simulink model "Model_silnika_mdl2"  (Simulink 9.1)
settings: Solver=ode45  StartTime=0.0  StopTime=100  FixedStep=1  RelTol=1e-8  EnableMultiTasking=on
values from neighbouring files (symbols this model uses):
  G = 4.2    [net_opuznienie_30.mat]    (also in parametrySilnika.m)
  G1 = 4.2    [net_opuznienie_30.mat]    (also in parametrySilnika.m)
  J = 1    [net_opuznienie_30.mat]    (also in parametrySilnika.m)
  J1 = 1.3    [net_opuznienie_30.mat]    (also in parametrySilnika.m = 1)
  Lt = 46    [net_opuznienie_30.mat]    (also in parametrySilnika.m)
  Lt1 = 59.8    [net_opuznienie_30.mat]    (also in parametrySilnika.m = 69)
  Lw = 125    [net_opuznienie_30.mat]    (also in parametrySilnika.m)
  Lw1 = 162.5    [net_opuznienie_30.mat]    (also in parametrySilnika.m = 125)
  Rt = 5    [net_opuznienie_30.mat]    (also in parametrySilnika.m)
  Rt1 = 5    [net_opuznienie_30.mat]    (also in parametrySilnika.m)
undefined symbols (not defined in the file or in its folder): sigbuilder_block
libraries: simulink x2
settings Model: Creator=zen  LastModifiedBy=Szwank
settings DataIOCC: LimitDataPoints=on  SignalLoggingSaveFormat=ModelDataLogs
settings OptimizationCC: ExpressionDepthLimit=2147483647  InitFltsAndDblsToZero=on
settings DebuggingCC: SaveWithParameterizedLinksMsg=none  SignalResolutionControl=TryResolveAllWithWarning  SolverPrmCheckMsg=warning  MultiTaskDSMMsg=warning  MultiTaskCondExecSysMsg=none  FcnCallInpInsideContextMsg=warning  StateNameClashWarn=warning
settings GRTTargetCC: TargetFcnLib=ansi_tfl_tmw.mat  GeneratePreprocessorConditionals=Disable all

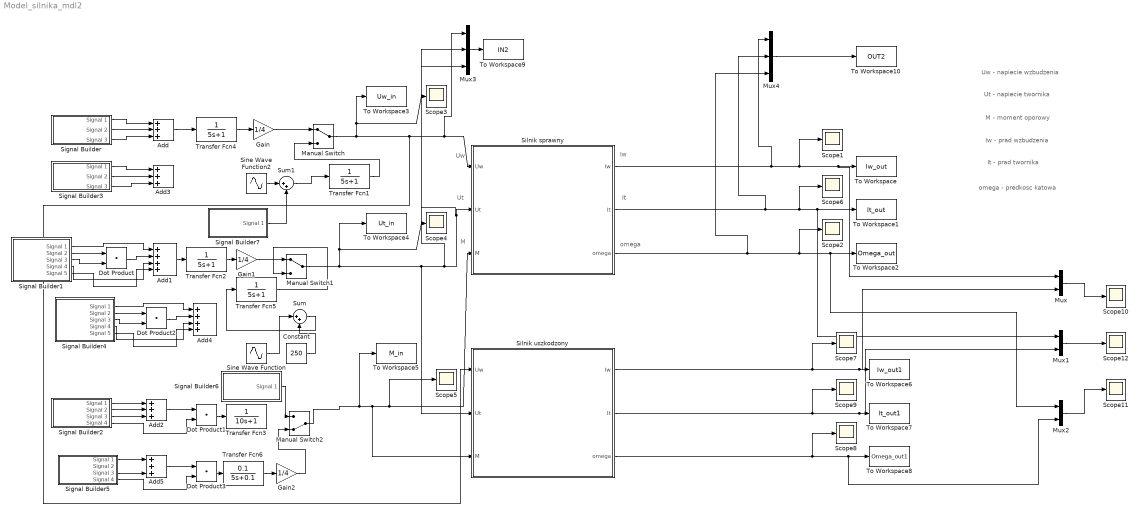
== system Model_silnika_mdl2 ==
  note: Uw
  note: Ut
  note: M
  note: Iw
  note: It
  note: omega
  note: Uw - napiecie wzbudzenia
  note: Ut - napiecie twornika
  note: M - moment oporowy
  note: Iw - prad wzbudzenia
  note: It - prad twornika
  note: omega - predkosc katowa
  Add{,2..3,5} (4 alike) : Sum  Inputs=+++
  Add1 : Sum  Inputs=++++
  Add4 : Sum  Inputs=++++
  Constant : Constant  Value=250
  Dot Product{,1..3} (4 alike) : DotProduct  InputSameDT=on  OutDataTypeStr=Inherit: Inherit via internal rule
  Gain : Gain  Gain=1/4
  Gain1 : Gain  Gain=1/4
  Gain2 : Gain  Gain=1/4
  Manual Switch : ManualSwitch
  Manual Switch1 : ManualSwitch
  Manual Switch2 : ManualSwitch  CurrentSetting=0
  Mux : Mux  Inputs=2
  Mux1 : Mux  Inputs=2
  Mux2 : Mux  Inputs=2
  Mux3 : Mux  Inputs=3
  Mux4 : Mux  Inputs=3
  Scope{1..12} (12 alike) : Scope
  Signal Builder : Subsystem  Tag=STV Subsys  LoadFcn=sigbuilder_block('load');  StartFcn=sigbuilder_block('start');  StopFcn=sigbuilder_block('stop');  ClipboardFcn=sigbuilder_block('clipboard');  mask(Sigbuilder block){tuvar=[0:10]}
      mask help: Create and generate interchangeable groups of signals whose waveforms are piecewise linear.
      mask init:
      | if ~strcmp(get_param(bdroot(gcbh),'SimulationStatus'),'stopped') tuvar = sigbuilder_block('maskInit'); end
      settings: CopyFcn=sigbuilder_block('copy');  DeleteFcn=sigbuilder_block('delete');  ModelCloseFcn=sigbuilder_block('modelClose');  PreSaveFcn=sigbuilder_block('preSave');  PauseFcn=sigbuilder_block('pause')  ContinueFcn=sigbuilder_block('continue')  NameChangeFcn=sigbuilder_block('namechange');  OpenFcn=sigbuilder_block('open',[159 116.25 948 506.25 ]);  CloseFcn=sigbuilder_block('close');
      mask Display: plot(0, 0, 100, 100,[2, 2, 32, 32, 2], [68, 8, 8, 68, 68],[32, 2], [38, 38], [32, 19, 2],[53, 60, 44], [32, 17, 17, 2],[16, 16, 31, 31]);txt = getActiveGroup(gcbh);text(2, 100, txt,'verticalAlignment', 'top');
  Signal Builder1 : Subsystem  Tag=STV Subsys  LoadFcn=sigbuilder_block('load');  StartFcn=sigbuilder_block('start');  StopFcn=sigbuilder_block('stop');  ClipboardFcn=sigbuilder_block('clipboard');  mask(Sigbuilder block){tuvar=[0:10]}
      mask help: Create and generate interchangeable groups of signals whose waveforms are piecewise linear.
      mask init:
      | if ~strcmp(get_param(bdroot(gcbh),'SimulationStatus'),'stopped') tuvar = sigbuilder_block('maskInit'); end
      settings: CopyFcn=sigbuilder_block('copy');  DeleteFcn=sigbuilder_block('delete');  ModelCloseFcn=sigbuilder_block('modelClose');  PreSaveFcn=sigbuilder_block('preSave');  PauseFcn=sigbuilder_block('pause')  ContinueFcn=sigbuilder_block('continue')  NameChangeFcn=sigbuilder_block('namechange');  OpenFcn=sigbuilder_block('open',[49.5 13.5 1254 711.75 ]);  CloseFcn=sigbuilder_block('close');
      mask Display: plot(0, 0, 100, 100,[2, 2, 32, 32, 2], [68, 8, 8, 68, 68],[32, 2], [38, 38], [32, 19, 2],[53, 60, 44], [32, 17, 17, 2],[16, 16, 31, 31]);txt = getActiveGroup(gcbh);text(2, 100, txt,'verticalAlignment', 'top');
  Signal Builder2 : Subsystem  Tag=STV Subsys  LoadFcn=sigbuilder_block('load');  StartFcn=sigbuilder_block('start');  StopFcn=sigbuilder_block('stop');  ClipboardFcn=sigbuilder_block('clipboard');  mask(Sigbuilder block){tuvar=[0:10]}
      mask help: Create and generate interchangeable groups of signals whose waveforms are piecewise linear.
      mask init:
      | if ~strcmp(get_param(bdroot(gcbh),'SimulationStatus'),'stopped') tuvar = sigbuilder_block('maskInit'); end
      settings: CopyFcn=sigbuilder_block('copy');  DeleteFcn=sigbuilder_block('delete');  ModelCloseFcn=sigbuilder_block('modelClose');  PreSaveFcn=sigbuilder_block('preSave');  PauseFcn=sigbuilder_block('pause')  ContinueFcn=sigbuilder_block('continue')  NameChangeFcn=sigbuilder_block('namechange');  OpenFcn=sigbuilder_block('open',[6 6 948 531 ]);  CloseFcn=sigbuilder_block('close');
      mask Display: plot(0, 0, 100, 100,[2, 2, 32, 32, 2], [68, 8, 8, 68, 68],[32, 2], [38, 38], [32, 19, 2],[53, 60, 44], [32, 17, 17, 2],[16, 16, 31, 31]);txt = getActiveGroup(gcbh);text(2, 100, txt,'verticalAlignment', 'top');
  Signal Builder3 : Subsystem  Tag=STV Subsys  LoadFcn=sigbuilder_block('load');  StartFcn=sigbuilder_block('start');  StopFcn=sigbuilder_block('stop');  ClipboardFcn=sigbuilder_block('clipboard');  mask(Sigbuilder block){tuvar=[0:10]}
      mask help: Create and generate interchangeable groups of signals whose waveforms are piecewise linear.
      mask init:
      | if ~strcmp(get_param(bdroot(gcbh),'SimulationStatus'),'stopped') tuvar = sigbuilder_block('maskInit'); end
      settings: CopyFcn=sigbuilder_block('copy');  DeleteFcn=sigbuilder_block('delete');  ModelCloseFcn=sigbuilder_block('modelClose');  PreSaveFcn=sigbuilder_block('preSave');  PauseFcn=sigbuilder_block('pause')  ContinueFcn=sigbuilder_block('continue')  NameChangeFcn=sigbuilder_block('namechange');  OpenFcn=sigbuilder_block('open',[6 30.75 948 506.25 ]);  CloseFcn=sigbuilder_block('close');
      mask Display: plot(0, 0, 100, 100,[2, 2, 32, 32, 2], [68, 8, 8, 68, 68],[32, 2], [38, 38], [32, 19, 2],[53, 60, 44], [32, 17, 17, 2],[16, 16, 31, 31]);txt = getActiveGroup(gcbh);text(2, 100, txt,'verticalAlignment', 'top');
  Signal Builder4 : Subsystem  Tag=STV Subsys  LoadFcn=sigbuilder_block('load');  StartFcn=sigbuilder_block('start');  StopFcn=sigbuilder_block('stop');  ClipboardFcn=sigbuilder_block('clipboard');  mask(Sigbuilder block){tuvar=[0:10]}
      mask help: Create and generate interchangeable groups of signals whose waveforms are piecewise linear.
      mask init:
      | if ~strcmp(get_param(bdroot(gcbh),'SimulationStatus'),'stopped') tuvar = sigbuilder_block('maskInit'); end
      settings: CopyFcn=sigbuilder_block('copy');  DeleteFcn=sigbuilder_block('delete');  ModelCloseFcn=sigbuilder_block('modelClose');  PreSaveFcn=sigbuilder_block('preSave');  PauseFcn=sigbuilder_block('pause')  ContinueFcn=sigbuilder_block('continue')  NameChangeFcn=sigbuilder_block('namechange');  OpenFcn=sigbuilder_block('open',[196.5 116.25 948 526.5 ]);  CloseFcn=sigbuilder_block('close');
      mask Display: plot(0, 0, 100, 100,[2, 2, 32, 32, 2], [68, 8, 8, 68, 68],[32, 2], [38, 38], [32, 19, 2],[53, 60, 44], [32, 17, 17, 2],[16, 16, 31, 31]);txt = getActiveGroup(gcbh);text(2, 100, txt,'verticalAlignment', 'top');
  Signal Builder5 : Subsystem  Tag=STV Subsys  LoadFcn=sigbuilder_block('load');  StartFcn=sigbuilder_block('start');  StopFcn=sigbuilder_block('stop');  ClipboardFcn=sigbuilder_block('clipboard');  mask(Sigbuilder block){tuvar=[0:10]}
      mask help: Create and generate interchangeable groups of signals whose waveforms are piecewise linear.
      mask init:
      | if ~strcmp(get_param(bdroot(gcbh),'SimulationStatus'),'stopped') tuvar = sigbuilder_block('maskInit'); end
      settings: CopyFcn=sigbuilder_block('copy');  DeleteFcn=sigbuilder_block('delete');  ModelCloseFcn=sigbuilder_block('modelClose');  PreSaveFcn=sigbuilder_block('preSave');  PauseFcn=sigbuilder_block('pause')  ContinueFcn=sigbuilder_block('continue')  NameChangeFcn=sigbuilder_block('namechange');  OpenFcn=sigbuilder_block('open',[57 31.5 948 531 ]);  CloseFcn=sigbuilder_block('close');
      mask Display: plot(0, 0, 100, 100,[2, 2, 32, 32, 2], [68, 8, 8, 68, 68],[32, 2], [38, 38], [32, 19, 2],[53, 60, 44], [32, 17, 17, 2],[16, 16, 31, 31]);txt = getActiveGroup(gcbh);text(2, 100, txt,'verticalAlignment', 'top');
  Signal Builder6 : Subsystem  Tag=STV Subsys  LoadFcn=sigbuilder_block('load');  StartFcn=sigbuilder_block('start');  StopFcn=sigbuilder_block('stop');  ClipboardFcn=sigbuilder_block('clipboard');  mask(Sigbuilder block){tuvar=[0:10]}
      mask help: Simulink:masks:SigbuilderBlock_MD
      mask init:
      | if ~strcmp(get_param(bdroot(gcbh),'SimulationStatus'),'stopped') tuvar = sigbuilder_block('maskInit'); end
      settings: CopyFcn=sigbuilder_block('copy');  DeleteFcn=sigbuilder_block('delete');  ModelCloseFcn=sigbuilder_block('modelClose');  PreSaveFcn=sigbuilder_block('preSave');  PauseFcn=sigbuilder_block('pause');  ContinueFcn=sigbuilder_block('continue');  NameChangeFcn=sigbuilder_block('namechange');  OpenFcn=sigbuilder_block('open',[437.6 199.2 550.4 400 ]);  CloseFcn=sigbuilder_block('close');
      mask Display: plot(0, 0, 100, 100,[2, 2, 32, 32, 2], [68, 8, 8, 68, 68],[32, 2], [38, 38], [32, 19, 2],[53, 60, 44], [32, 17, 17, 2],[16, 16, 31, 31]);txt = getActiveGroup(gcbh);text(2, 100, txt,'verticalAlignment', 'top');
  Signal Builder7 : Subsystem  Tag=STV Subsys  LoadFcn=sigbuilder_block('load');  StartFcn=sigbuilder_block('start');  StopFcn=sigbuilder_block('stop');  ClipboardFcn=sigbuilder_block('clipboard');  mask(Sigbuilder block){tuvar=[0:10]}
      mask help: Simulink:masks:SigbuilderBlock_MD
      mask init:
      | if ~strcmp(get_param(bdroot(gcbh),'SimulationStatus'),'stopped') tuvar = sigbuilder_block('maskInit'); end
      settings: CopyFcn=sigbuilder_block('copy');  DeleteFcn=sigbuilder_block('delete');  ModelCloseFcn=sigbuilder_block('modelClose');  PreSaveFcn=sigbuilder_block('preSave');  PauseFcn=sigbuilder_block('pause');  ContinueFcn=sigbuilder_block('continue');  NameChangeFcn=sigbuilder_block('namechange');  OpenFcn=sigbuilder_block('open',[437.6 199.2 550.4 400 ]);  CloseFcn=sigbuilder_block('close');
      mask Display: plot(0, 0, 100, 100,[2, 2, 32, 32, 2], [68, 8, 8, 68, 68],[32, 2], [38, 38], [32, 19, 2],[53, 60, 44], [32, 17, 17, 2],[16, 16, 31, 31]);txt = getActiveGroup(gcbh);text(2, 100, txt,'verticalAlignment', 'top');
  Silnik sprawny : Subsystem
  Silnik uszkodzony : Subsystem
  Sine Wave Function : Sin  Amplitude=30  Frequency=0.3  SampleTime=0
  Sine Wave Function2 : Sin  Amplitude=20  Frequency=0.1  Phase=pi/2  SampleTime=0
  Sum : Sum  Inputs=|++
  Sum1 : Sum  Inputs=|++
  To Workspace : ToWorkspace  VariableName=Iw_out  SaveFormat=Structure With Time  SampleTime=0.25
  To Workspace1 : ToWorkspace  VariableName=It_out  SaveFormat=Structure With Time  SampleTime=0.25
  To Workspace10 : ToWorkspace  VariableName=OUT2  SampleTime=0.1
      settings: Save2DSignal=2-D array (concatenate along first dimension)
  To Workspace2 : ToWorkspace  VariableName=Omega_out  SaveFormat=Structure With Time  SampleTime=0.25
  To Workspace3 : ToWorkspace  VariableName=Uw_in  SaveFormat=Structure With Time  SampleTime=0.25
  To Workspace4 : ToWorkspace  VariableName=Ut_in  SaveFormat=Structure With Time  SampleTime=0.25
  To Workspace5 : ToWorkspace  VariableName=M_in  SaveFormat=Structure With Time  SampleTime=0.25
  To Workspace6 : ToWorkspace  VariableName=Iw_out1  SaveFormat=Structure With Time  SampleTime=0.25
  To Workspace7 : ToWorkspace  VariableName=It_out1  SaveFormat=Structure With Time  SampleTime=0.25
  To Workspace8 : ToWorkspace  VariableName=Omega_out1  SaveFormat=Structure With Time  SampleTime=0.25
  To Workspace9 : ToWorkspace  VariableName=IN2  SampleTime=0.1
      settings: Save2DSignal=2-D array (concatenate along first dimension)
  Transfer Fcn{1..2,4..5} (4 alike) : TransferFcn  Denominator=[5 1]
  Transfer Fcn3 : TransferFcn  Denominator=[10 1]
  Transfer Fcn6 : TransferFcn  Numerator=[0.1]  Denominator=[5 0.1]
  wires:
  Add/1 -> Transfer Fcn4/1
  Signal Builder1/2(Signal 2) -> Dot Product/1
  Signal Builder1/3(Signal 3) -> Dot Product/2
  Add2/1 -> Dot Product1/1
  Dot Product1/1 -> Transfer Fcn3/1
  Signal Builder/1(Signal 1) -> Add/1
  Signal Builder/2(Signal 2) -> Add/2
  Signal Builder/3(Signal 3) -> Add/3
  Signal Builder1/1(Signal 1) -> Add1/1
  Dot Product/1 -> Add1/2
  Signal Builder1/4(Signal 4) -> Add1/3
  Signal Builder1/5(Signal 5) -> Add1/4
  Add1/1 -> Transfer Fcn2/1
  Signal Builder2/1(Signal 1) -> Add2/1
  Signal Builder2/2(Signal 2) -> Add2/2
  Signal Builder2/3(Signal 3) -> Add2/3
  Signal Builder2/4(Signal 4) -> Dot Product1/2
  Signal Builder3/1(Signal 1) -> Add3/1
  Signal Builder4/2(Signal 2) -> Dot Product2/1
  Signal Builder4/3(Signal 3) -> Dot Product2/2
  Signal Builder4/1(Signal 1) -> Add4/1
  Dot Product2/1 -> Add4/2
  Signal Builder4/4(Signal 4) -> Add4/3
  Signal Builder4/5(Signal 5) -> Add4/4
  Manual Switch2/1 -> To Workspace5/1, Silnik uszkodzony/3(M), Scope5/1, Silnik sprawny/3(M)
  Add5/1 -> Dot Product3/1
  Dot Product3/1 -> Transfer Fcn6/1
  Signal Builder5/1(Signal 1) -> Add5/1
  Signal Builder5/3(Signal 3) -> Add5/3
  Signal Builder5/4(Signal 4) -> Dot Product3/2
  Manual Switch/1 -> To Workspace3/1, Scope3/1, Silnik uszkodzony/1(Uw), Mux3/1, Silnik sprawny/1(Uw)
  Signal Builder3/2(Signal 2) -> Add3/2
  Signal Builder3/3(Signal 3) -> Add3/3
  Silnik uszkodzony/1(Iw) -> Scope7/1, Mux/2, To Workspace6/1
  Silnik uszkodzony/2(It) -> Scope9/1, Mux1/2, To Workspace7/1
  Silnik uszkodzony/3(omega) -> Scope8/1, Mux2/2, To Workspace8/1
  Mux/1 -> Scope10/1
  Mux1/1 -> Scope12/1
  Mux2/1 -> Scope11/1
  Signal Builder6/1(Signal 1) -> Manual Switch2/1
  Sine Wave Function/1 -> Sum/1
  Constant/1 -> Sum/2
  Sine Wave Function2/1 -> Sum1/1
  Sum1/1 -> Transfer Fcn1/1
  Transfer Fcn1/1 -> Manual Switch/2
  Transfer Fcn5/1 -> Manual Switch1/2
  Sum/1 -> Transfer Fcn5/1
  Signal Builder7/1(Signal 1) -> Sum1/2
  Mux3/1 -> To Workspace9/1
  Manual Switch1/1 -> To Workspace4/1, Scope4/1, Silnik uszkodzony/2(Ut), Mux3/3, Mux3/2, Silnik sprawny/2(Ut)
  Silnik sprawny/2(It) -> Mux4/2, To Workspace1/1, Mux1/1, Scope6/1
  Silnik sprawny/1(Iw) -> Mux4/1, Mux/1, To Workspace/1, Scope1/1
  Silnik sprawny/3(omega) -> Mux4/3, Mux2/1, To Workspace2/1, Scope2/1
  Transfer Fcn4/1 -> Gain/1
  Gain/1 -> Manual Switch/1
  Transfer Fcn2/1 -> Gain1/1
  Gain1/1 -> Manual Switch1/1
  Transfer Fcn6/1 -> Gain2/1
  Gain2/1 -> Manual Switch2/2
  Mux4/1 -> To Workspace10/1

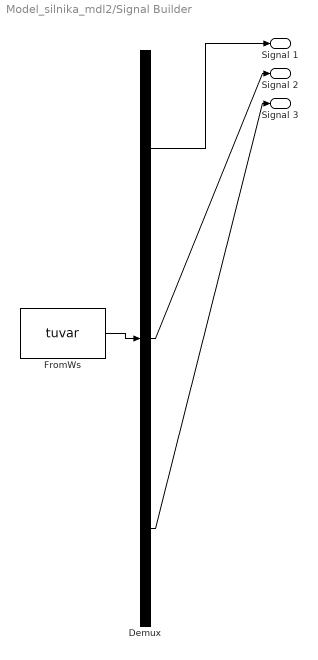
== system Model_silnika_mdl2/Signal Builder ==
  Demux : Demux  Tag=STV Demux  Outputs=3
  FromWs : FromWorkspace  Tag=STV FromWs  VariableName=tuvar  SampleTime=0  SigBuilderData=DataTag0  VnvData=DataTag1
      SigBuilderData=|
      | common.afterFinalStr = 'Extrapolate'
      | common.sampleTime = 0
      | dataSet.timeRange = [0 3000]
      | dataSet.name = 'Group 1'
      | sbobj.Groups.Name = 'Group 1'
      | sbobj.Groups.Signals(1).Name = 'Signal 1'
      | sbobj.Groups.Signals(1).XData = [0 275 275 425 850 850 3000]
      | sbobj.Groups.Signals(1).YData = [230 230 229.5 229.5 229.5 230.2 230]
      | sbobj.Groups.Signals(2).Name = 'Signal 2'
      | sbobj.Groups.Signals(2).XData = [0 12.5 25 37.5 50 62.5 75 87.5 100 112.5 125 137.5 150 162.5 175 187.5 200 212.5 225 237.5 250 262.5 275 287.5 300 312.5 325 337.5 350 362.5 375 387.5 400 412.5 425 437.5 450 462.5 475 487.5 500 512.5 525 537.5 550 562.5 575 587.5 600 612.5 625 637.5 650 662.5 675 687.5 700 712.5 725 737.5 750 762.5 775 787.5 800 812.5 825 837.5 850 862.5 875 887.5 900 912.5 925 937.5 950 962.5 975 987.5 1000 1012.5 1025 1037.5 1050 1062.5 1075 1087.5 1100 1112.5 1125 1137.5 1150 1162.5 1175 1187.5 1200 1212.5 1225 1237.5 1250 1262.5 1275 1287.5 1300 1312.5 1325 1337.5 1350 1362.5 1375 1387.5 1400 1412.5 1425 1437.5 1450 1462.5 1475 1487.5 1500 1512.5 1525 1537.5 1550 1562.5 1575 1587.5 1600 1612.5 1625 1637.5 1650 1662.5 1675 1687.5 1700 1712.5 1725 1737.5 1750 1762.5 1775 1787.5 1800 1812.5 1825 1837.5 1850 1862.5 1875 1887.5 1900 1912.5 1925 1937.5 1950 1962.5 1975 1987.5 2000 2012.5 2025 2037.5 2050 2062.5 2075 2087.5 2100 2112.5 2125 2137.5 2150 2162.5 2175 2187.5 2200 2212.5 2225 2237.5 2250 2262.5 2275 2287.5 2300 2312.5 2325 2337.5 2350 2362.5 2375 2387.5 2400 2412.5 2425 2437.5 2450 2462.5 2475 2487.5 2500 2512.5 2525 2537.5 2550 2562.5 2575 2587.5 2600 2612.5 2625 2637.5 2650 2662.5 2675 2687.5 2700 2712.5 2725 2737.5 2750 2762.5 2775 2787.5 2800 2812.5 2825 2837.5 2850 2862.5 2875 2887.5 2900 2912.5 2925 2937.5 2950 2962.5 2975 2987.5 3000]
      | sbobj.Groups.Signals(2).YData = [0 10.6066017178 15 10.6066017178 1.83697019872e-15 -10.6066017178 -15 -10.6066017178 0 10.6066017178 15 10.6066017178 ... (241 elements, 1x241)]
      | sbobj.Groups.Signals(3).Name = 'Signal 3'
      | sbobj.Groups.Signals(3).XData = [0 200 200 240 240 280 280 360 360 400 400 520 520 640 640 840 840 1040 1040 1080 1080 1160 1160 1200 1200 1280 1280 1360 1360 1520 1520 1560 1560 1640 1640 1720 1720 1880 1880 1960 1960 2000 2000 2040 2040 2080 2080 2200 2200 2240 2240 2280 2280 2520 2520 2600 2600 2760 2760 2800 2800 2880 2880 3000]
      | sbobj.Groups.Signals(3).YData = [5 5 -5 -5 5 5 -5 -5 5 5 -5 -5 5 5 -5 -5 5 5 -5 -5 5 5 -5 -5 5 5 -5 -5 5 5 -5 -5 5 5 -5 -5 5 5 -5 -5 5 5 -5 -5 5 5 -5 -5 5 5 -5 -5 5 5 -5 -5 5 5 -5 -5 5 5 -5 -5]
      | sbobj.Groups.TimeRange = [0 3000]
  Signal 1 : Outport  Tag=STV Outport
  Signal 2 : Outport  Tag=STV Outport  Port=2
  Signal 3 : Outport  Tag=STV Outport  Port=3
  wires:
  Demux/1 -> Signal 1/1
  FromWs/1 -> Demux/1
  Demux/2 -> Signal 2/1
  Demux/3 -> Signal 3/1

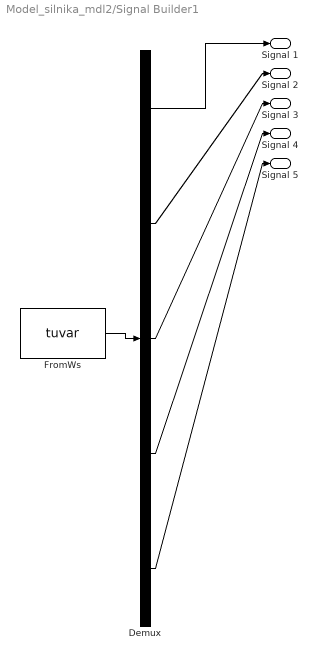
== system Model_silnika_mdl2/Signal Builder1 ==
  Demux : Demux  Tag=STV Demux  Outputs=5
  FromWs : FromWorkspace  Tag=STV FromWs  VariableName=tuvar  SampleTime=0  SigBuilderData=DataTag2  VnvData=DataTag3
      SigBuilderData=|
      | common.afterFinalStr = 'Extrapolate'
      | common.sampleTime = 0
      | dataSet.timeRange = [0 3000]
      | dataSet.name = 'Group 1'
      | sbobj.Groups.Name = 'Group 1'
      | sbobj.Groups.Signals(1).Name = 'Signal 1'
      | sbobj.Groups.Signals(1).XData = [0 240 250 3000]
      | sbobj.Groups.Signals(1).YData = [0 231 230 230]
      | sbobj.Groups.Signals(2).Name = 'Signal 2'
      | sbobj.Groups.Signals(2).XData = [0 6.25 12.5 18.75 25 31.25 37.5 43.75 50 56.25 62.5 68.75 ... (481 elements, 1x481)]
      | sbobj.Groups.Signals(2).YData = [0 1.41421356237 2 1.41421356237 -0.15 -1.41421356237 -2 -1.41421356237 0 1.41421356237 2 1.41421356237 ... (481 elements, 1x481)]
      | sbobj.Groups.Signals(3).Name = 'Signal 3'
      | sbobj.Groups.Signals(3).XData = [0 240 240 1000 3000]
      | sbobj.Groups.Signals(3).YData = [0 0 0.0085 0 0]
      | sbobj.Groups.Signals(4).Name = 'Signal 4'
      | sbobj.Groups.Signals(4).XData = [0 25 50 75 100 125 150 175 200 225 250 275 300 325 350 375 400 425 450 475 500 525 550 575 600 625 650 675 700 725 750 775 800 825 850 875 900 925 950 975 1000 1025 1050 1075 1100 1125 1150 1175 1200 1225 1250 1275 1300 1325 1350 1375 1400 1425 1450 1475 1500 1525 1550 1575 1600 1625 1650 1675 1700 1725 1750 1775 1800 1825 1850 1875 1900 1925 1950 1975 2000 2025 2050 2075 2100 2125 2150 2175 2200 2225 2250 2275 2300 2325 2350 2375 2400 2425 2450 2475 2500 2525 2550 2575 2600 2625 2650 2675 2700 2725 2750 2775 2800 2825 2850 2875 2900 2925 2950 2975 3000]
      | sbobj.Groups.Signals(4).YData = [0 3.53553390593 5 3.53553390593 6.12323399574e-16 -3.53553390593 -5 -3.53553390593 0 3.53553390593 5 3.53553390593 6.12323399574e-16 -3.53553390593 -5 -3.53553390593 0 3.53553390593 5 3.53553390593 6.12323399574e-16 -3.53553390593 -5 -3.53553390593 0 3.53553390593 5 3.53553390593 6.12323399574e-16 -3.53553390593 -5 -3.53553390593 0 3.53553390593 5 3.53553390593 6.12323399574e-16 -3.53553390593 -5 -3.53553390593 0 3.53553390593 5 3.53553390593 6.12323399574e-16 -3.53553390593 -5 -3.53553390593 0 3.53553390593 5 3.53553390593 6.12323399574e-16 -3.53553390593 -5 -3.53553390593 0 3.53553390593 5 3.53553390593 6.12323399574e-16 -3.53553390593 -5 -3.53553390593 0 3.53553390593 5 3.53553390593 6.12323399574e-16 -3.53553390593 -5 -3.53553390593 0 3.53553390593 5 3.53553390593 6.12323399574e-16 -3.53553390593 -5 -3.53553390593 0 3.53553390593 5 3.53553390593 6.12323399574e-16 -3.53553390593 -5 -3.53553390593 0 3.53553390593 5 3.53553390593 6.12323399574e-16 -3.53553390593 -5 -3.53553390593 0 3.53553390593 5 3.53553390593 6.12323399574e-16 -3.53553390593 -5 -3.53553390593 0 3.53553390593 5 3.53553390593 6.12323399574e-16 -3.53553390593 -5 -3.53553390593 0 3.53553390593 5 3.53553390593 6.12323399574e-16 -3.53553390593 -5 -3.53553390593 0]
      | sbobj.Groups.Signals(5).Name = 'Signal 5'
      | sbobj.Groups.Signals(5).XData = [0 125 125 250 250 375 375 625 625 750 750 1125 1125 1375 1375 1500 1500 1875 1875 2375 2375 2750 2750 2875 2875 3000]
      | sbobj.Groups.Signals(5).YData = [7.8 7.8 8 8 -8 -8 8 8 -8 -8 8 8 -8 -8 8 8 -8 -8 8 8 -8 -8 8 8 -8 -8]
      | sbobj.Groups.TimeRange = [0 3000]
  Signal 1 : Outport  Tag=STV Outport
  Signal 2 : Outport  Tag=STV Outport  Port=2
  Signal 3 : Outport  Tag=STV Outport  Port=3
  Signal 4 : Outport  Tag=STV Outport  Port=4
  Signal 5 : Outport  Tag=STV Outport  Port=5
  wires:
  FromWs/1 -> Demux/1
  Demux/1 -> Signal 1/1
  Demux/2 -> Signal 2/1
  Demux/3 -> Signal 3/1
  Demux/4 -> Signal 4/1
  Demux/5 -> Signal 5/1

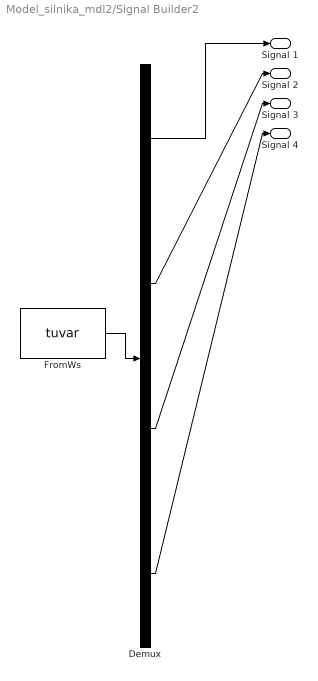
== system Model_silnika_mdl2/Signal Builder2 ==
  Demux : Demux  Tag=STV Demux
  FromWs : FromWorkspace  Tag=STV FromWs  VariableName=tuvar  SampleTime=0  SigBuilderData=DataTag4  VnvData=DataTag5
      SigBuilderData=|
      | common.afterFinalStr = 'Extrapolate'
      | common.sampleTime = 0
      | dataSet.timeRange = [0 3000]
      | dataSet.name = 'Group 1'
      | sbobj.Groups.Name = 'Group 1'
      | sbobj.Groups.Signals(1).Name = 'Signal 1'
      | sbobj.Groups.Signals(1).XData = [0 242 242 1002 1002 1227 1227 1604 1604 2163 2163 2441 2441 2870 2870 3000]
      | sbobj.Groups.Signals(1).YData = [0 0 1.3 1.3 0.8 0.8 1.95 1.95 2.8 2.8 3.5 3.5 4.5 4.5 5.2 5.2]
      | sbobj.Groups.Signals(2).Name = 'Signal 2'
      | sbobj.Groups.Signals(2).XData = [0 1.5625 3.125 4.6875 6.25 7.8125 9.375 10.9375 12.5 14.0625 15.625 17.1875 ... (1921 elements, 1x1921)]
      | sbobj.Groups.Signals(2).YData = [0 0.141421356237 0.2 0.141421356237 2.44929359829e-17 -0.141421356237 -0.2 -0.141421356237 0 0.141421356237 0.2 0.141421356237 ... (1921 elements, 1x1921)]
      | sbobj.Groups.Signals(3).Name = 'Signal 3'
      | sbobj.Groups.Signals(3).XData = [0 295 295 500 500 833.333333333 833.333333333 1500 1500 1666.66666667 1666.66666667 1833.33333333 1833.33333333 2000 2000 2666.66666667 2666.66666667 2833.33333333 2833.33333333 3000]
      | sbobj.Groups.Signals(3).YData = [0.2 0.2 1 1 1.5 1.5 0 0 1.5 1.5 0 0 1.5 1.5 0 0 1.5 1.5 0 0]
      | sbobj.Groups.Signals(4).Name = 'Signal 4'
      | sbobj.Groups.Signals(4).XData = [0 302 302 3000]
      | sbobj.Groups.Signals(4).YData = [0 0 1 1]
      | sbobj.Groups.TimeRange = [0 3000]
  Signal 1 : Outport  Tag=STV Outport
  Signal 2 : Outport  Tag=STV Outport  Port=2
  Signal 3 : Outport  Tag=STV Outport  Port=3
  Signal 4 : Outport  Tag=STV Outport  Port=4
  wires:
  Demux/3 -> Signal 3/1
  Demux/2 -> Signal 2/1
  FromWs/1 -> Demux/1
  Demux/1 -> Signal 1/1
  Demux/4 -> Signal 4/1

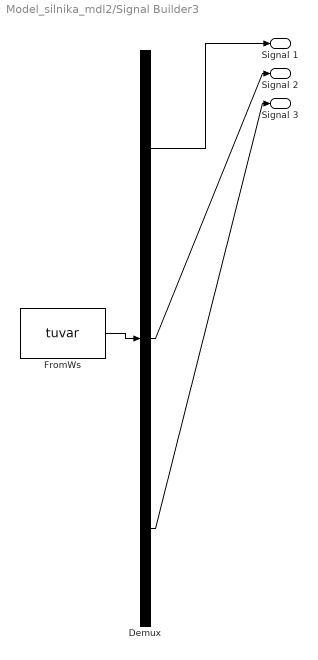
== system Model_silnika_mdl2/Signal Builder3 ==
  Demux : Demux  Tag=STV Demux  Outputs=3
  FromWs : FromWorkspace  Tag=STV FromWs  VariableName=tuvar  SampleTime=0  SigBuilderData=DataTag6  VnvData=DataTag7
      SigBuilderData=|
      | common.afterFinalStr = 'Extrapolate'
      | common.sampleTime = 0
      | dataSet.timeRange = [0 3000]
      | dataSet.name = 'Group 1'
      | sbobj.Groups.Name = 'Group 1'
      | sbobj.Groups.Signals(1).Name = 'Signal 1'
      | sbobj.Groups.Signals(1).XData = [0 275 755 850 3000]
      | sbobj.Groups.Signals(1).YData = [400 400 400 400 400]
      | sbobj.Groups.Signals(2).Name = 'Signal 2'
      | sbobj.Groups.Signals(2).XData = [0 12.5 25 37.5 50 62.5 75 87.5 100 112.5 125 137.5 150 162.5 175 187.5 200 212.5 225 237.5 250 262.5 275 287.5 300 312.5 325 337.5 350 362.5 375 387.5 400 412.5 425 437.5 450 462.5 475 487.5 500 512.5 525 537.5 550 562.5 575 587.5 600 612.5 625 637.5 650 662.5 675 687.5 700 712.5 725 737.5 750 762.5 775 787.5 800 812.5 825 837.5 850 862.5 875 887.5 900 912.5 925 937.5 950 962.5 975 987.5 1000 1012.5 1025 1037.5 1050 1062.5 1075 1087.5 1100 1112.5 1125 1137.5 1150 1162.5 1175 1187.5 1200 1212.5 1225 1237.5 1250 1262.5 1275 1287.5 1300 1312.5 1325 1337.5 1350 1362.5 1375 1387.5 1400 1412.5 1425 1437.5 1450 1462.5 1475 1487.5 1500 1512.5 1525 1537.5 1550 1562.5 1575 1587.5 1600 1612.5 1625 1637.5 1650 1662.5 1675 1687.5 1700 1712.5 1725 1737.5 1750 1762.5 1775 1787.5 1800 1812.5 1825 1837.5 1850 1862.5 1875 1887.5 1900 1912.5 1925 1937.5 1950 1962.5 1975 1987.5 2000 2012.5 2025 2037.5 2050 2062.5 2075 2087.5 2100 2112.5 2125 2137.5 2150 2162.5 2175 2187.5 2200 2212.5 2225 2237.5 2250 2262.5 2275 2287.5 2300 2312.5 2325 2337.5 2350 2362.5 2375 2387.5 2400 2412.5 2425 2437.5 2450 2462.5 2475 2487.5 2500 2512.5 2525 2537.5 2550 2562.5 2575 2587.5 2600 2612.5 2625 2637.5 2650 2662.5 2675 2687.5 2700 2712.5 2725 2737.5 2750 2762.5 2775 2787.5 2800 2812.5 2825 2837.5 2850 2862.5 2875 2887.5 2900 2912.5 2925 2937.5 2950 2962.5 2975 2987.5 3000]
      | sbobj.Groups.Signals(2).YData = [0 10.6066017178 15 10.6066017178 1.83697019872e-15 -10.6066017178 -15 -10.6066017178 0 10.6066017178 15 10.6066017178 ... (241 elements, 1x241)]
      | sbobj.Groups.Signals(3).Name = 'Signal 3'
      | sbobj.Groups.Signals(3).XData = [0 200 200 240 240 280 280 360 360 400 400 520 520 640 640 840 840 1040 1040 1080 1080 1160 1160 1200 1200 1280 1280 1360 1360 1520 1520 1560 1560 1640 1640 1720 1720 1880 1880 1960 1960 2000 2000 2040 2040 2080 2080 2200 2200 2240 2240 2280 2280 2520 2520 2600 2600 2760 2760 2800 2800 2880 2880 3000]
      | sbobj.Groups.Signals(3).YData = [5 5 -5 -5 5 5 -5 -5 5 5 -5 -5 5 5 -5 -5 5 5 -5 -5 5 5 -5 -5 5 5 -5 -5 5 5 -5 -5 5 5 -5 -5 5 5 -5 -5 5 5 -5 -5 5 5 -5 -5 5 5 -5 -5 5 5 -5 -5 5 5 -5 -5 5 5 -5 -5]
      | sbobj.Groups.TimeRange = [0 3000]
  Signal 1 : Outport  Tag=STV Outport
  Signal 2 : Outport  Tag=STV Outport  Port=2
  Signal 3 : Outport  Tag=STV Outport  Port=3
  wires:
  Demux/3 -> Signal 3/1
  Demux/2 -> Signal 2/1
  FromWs/1 -> Demux/1
  Demux/1 -> Signal 1/1

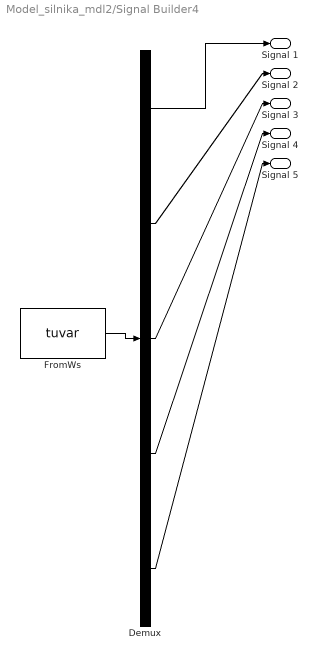
== system Model_silnika_mdl2/Signal Builder4 ==
  Demux : Demux  Tag=STV Demux  Outputs=5
  FromWs : FromWorkspace  Tag=STV FromWs  VariableName=tuvar  SampleTime=0  SigBuilderData=DataTag8  VnvData=DataTag9
      SigBuilderData=|
      | common.afterFinalStr = 'Extrapolate'
      | common.sampleTime = 0
      | dataSet.timeRange = [0 3000]
      | dataSet.name = 'Group 1'
      | sbobj.Groups.Name = 'Group 1'
      | sbobj.Groups.Signals(1).Name = 'Signal 1'
      | sbobj.Groups.Signals(1).XData = [0 240 250 3000]
      | sbobj.Groups.Signals(1).YData = [145 150 150 150]
      | sbobj.Groups.Signals(2).Name = 'Signal 2'
      | sbobj.Groups.Signals(2).XData = [0 6.25 12.5 18.75 25 31.25 37.5 43.75 50 56.25 62.5 68.75 ... (481 elements, 1x481)]
      | sbobj.Groups.Signals(2).YData = [0 1.41421356237 2 1.41421356237 -0.15 -1.41421356237 -2 -1.41421356237 0 1.41421356237 2 1.41421356237 ... (481 elements, 1x481)]
      | sbobj.Groups.Signals(3).Name = 'Signal 3'
      | sbobj.Groups.Signals(3).XData = [0 500 500 1500 3000]
      | sbobj.Groups.Signals(3).YData = [0 0 1 0 0]
      | sbobj.Groups.Signals(4).Name = 'Signal 4'
      | sbobj.Groups.Signals(4).XData = [0 25 50 75 100 125 150 175 200 225 250 275 300 325 350 375 400 425 450 475 500 525 550 575 600 625 650 675 700 725 750 775 800 825 850 875 900 925 950 975 1000 1025 1050 1075 1100 1125 1150 1175 1200 1225 1250 1275 1300 1325 1350 1375 1400 1425 1450 1475 1500 1525 1550 1575 1600 1625 1650 1675 1700 1725 1750 1775 1800 1825 1850 1875 1900 1925 1950 1975 2000 2025 2050 2075 2100 2125 2150 2175 2200 2225 2250 2275 2300 2325 2350 2375 2400 2425 2450 2475 2500 2525 2550 2575 2600 2625 2650 2675 2700 2725 2750 2775 2800 2825 2850 2875 2900 2925 2950 2975 3000]
      | sbobj.Groups.Signals(4).YData = [0 3.53553390593 5 3.53553390593 6.12323399574e-16 -3.53553390593 -5 -3.53553390593 0 3.53553390593 5 3.53553390593 6.12323399574e-16 -3.53553390593 -5 -3.53553390593 0 3.53553390593 5 3.53553390593 6.12323399574e-16 -3.53553390593 -5 -3.53553390593 0 3.53553390593 5 3.53553390593 6.12323399574e-16 -3.53553390593 -5 -3.53553390593 0 3.53553390593 5 3.53553390593 6.12323399574e-16 -3.53553390593 -5 -3.53553390593 0 3.53553390593 5 3.53553390593 6.12323399574e-16 -3.53553390593 -5 -3.53553390593 0 3.53553390593 5 3.53553390593 6.12323399574e-16 -3.53553390593 -5 -3.53553390593 0 3.53553390593 5 3.53553390593 6.12323399574e-16 -3.53553390593 -5 -3.53553390593 0 3.53553390593 5 3.53553390593 6.12323399574e-16 -3.53553390593 -5 -3.53553390593 0 3.53553390593 5 3.53553390593 6.12323399574e-16 -3.53553390593 -5 -3.53553390593 0 3.53553390593 5 3.53553390593 6.12323399574e-16 -3.53553390593 -5 -3.53553390593 0 3.53553390593 5 3.53553390593 6.12323399574e-16 -3.53553390593 -5 -3.53553390593 0 3.53553390593 5 3.53553390593 6.12323399574e-16 -3.53553390593 -5 -3.53553390593 0 3.53553390593 5 3.53553390593 6.12323399574e-16 -3.53553390593 -5 -3.53553390593 0 3.53553390593 5 3.53553390593 6.12323399574e-16 -3.53553390593 -5 -3.53553390593 0]
      | sbobj.Groups.Signals(5).Name = 'Signal 5'
      | sbobj.Groups.Signals(5).XData = [0 125 125 250 250 375 375 625 625 750 750 1125 1125 1375 1375 1500 1500 1875 1875 2375 2375 2750 2750 2875 2875 3000]
      | sbobj.Groups.Signals(5).YData = [7.8 7.8 8 8 -8 -8 8 8 -8 -8 8 8 -8 -8 8 8 -8 -8 8 8 -8 -8 8 8 -8 -8]
      | sbobj.Groups.TimeRange = [0 3000]
  Signal 1 : Outport  Tag=STV Outport
  Signal 2 : Outport  Tag=STV Outport  Port=2
  Signal 3 : Outport  Tag=STV Outport  Port=3
  Signal 4 : Outport  Tag=STV Outport  Port=4
  Signal 5 : Outport  Tag=STV Outport  Port=5
  wires:
  FromWs/1 -> Demux/1
  Demux/1 -> Signal 1/1
  Demux/2 -> Signal 2/1
  Demux/3 -> Signal 3/1
  Demux/4 -> Signal 4/1
  Demux/5 -> Signal 5/1

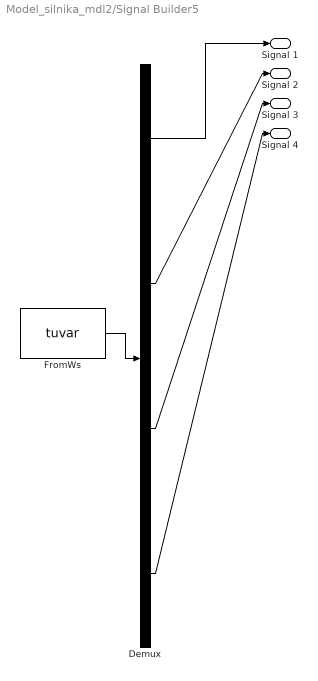
== system Model_silnika_mdl2/Signal Builder5 ==
  Demux : Demux  Tag=STV Demux
  FromWs : FromWorkspace  Tag=STV FromWs  VariableName=tuvar  SampleTime=0  SigBuilderData=DataTag10  VnvData=DataTag11
      SigBuilderData=|
      | common.afterFinalStr = 'Extrapolate'
      | common.sampleTime = 0
      | dataSet.timeRange = [0 3000]
      | dataSet.name = 'Group 1'
      | sbobj.Groups.Name = 'Group 1'
      | sbobj.Groups.Signals(1).Name = 'Signal 1'
      | sbobj.Groups.Signals(1).XData = [0 242 242 1002 1002 1227 1227 1604 1604 2163 2163 2441 2441 2870 2870 3000]
      | sbobj.Groups.Signals(1).YData = [0 0 1.3 1.3 0.8 0.8 1.95 1.95 2.8 2.8 3.5 3.5 4.5 4.5 5.2 5.2]
      | sbobj.Groups.Signals(2).Name = 'Signal 2'
      | sbobj.Groups.Signals(2).XData = [0 1.5625 3.125 4.6875 6.25 7.8125 9.375 10.9375 12.5 14.0625 15.625 17.1875 ... (1921 elements, 1x1921)]
      | sbobj.Groups.Signals(2).YData = [0 0.141421356237 0.2 0.141421356237 2.44929359829e-17 -0.141421356237 -0.2 -0.141421356237 0 0.141421356237 0.2 0.141421356237 ... (1921 elements, 1x1921)]
      | sbobj.Groups.Signals(3).Name = 'Signal 3'
      | sbobj.Groups.Signals(3).XData = [0 295 295 500 500 833.333333333 833.333333333 1500 1500 1666.66666667 1666.66666667 1833.33333333 1833.33333333 2000 2000 2666.66666667 2833.33333333 2833.33333333 3000]
      | sbobj.Groups.Signals(3).YData = [0.2 0.2 1 1 1.5 1.5 1.55 1.55 1.5 1.5 0 0 1.5 1.5 0 1.5 1.5 0 0]
      | sbobj.Groups.Signals(4).Name = 'Signal 4'
      | sbobj.Groups.Signals(4).XData = [0 302 3000]
      | sbobj.Groups.Signals(4).YData = [1.02 1 1]
      | sbobj.Groups.TimeRange = [0 3000]
  Signal 1 : Outport  Tag=STV Outport
  Signal 2 : Outport  Tag=STV Outport  Port=2
  Signal 3 : Outport  Tag=STV Outport  Port=3
  Signal 4 : Outport  Tag=STV Outport  Port=4
  wires:
  Demux/3 -> Signal 3/1
  Demux/2 -> Signal 2/1
  FromWs/1 -> Demux/1
  Demux/1 -> Signal 1/1
  Demux/4 -> Signal 4/1

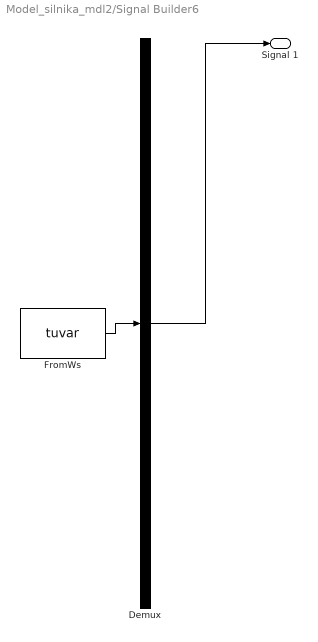
== system Model_silnika_mdl2/Signal Builder6 ==
  Demux : Demux  Tag=STV Demux  Outputs=1
  FromWs : FromWorkspace  Tag=STV FromWs  VariableName=tuvar  SampleTime=0  SigBuilderData=DataTag12  VnvData=DataTag13
      SigBuilderData=|
      | common.afterFinalStr = 'Extrapolate'
      | common.sampleTime = 0
      | dataSet.timeRange = [0 10]
      | dataSet.name = 'Group 1'
      | sbobj.Groups.Name = 'Group 1'
      | sbobj.Groups.Signals.Name = 'Signal 1'
      | sbobj.Groups.Signals.XData = [0 4 4 6 6 10]
      | sbobj.Groups.Signals.YData = [0.205 0.4 0.11 0.61 0.325 0.225]
  Signal 1 : Outport  Tag=STV Outport
  wires:
  Demux/1 -> Signal 1/1
  FromWs/1 -> Demux/1

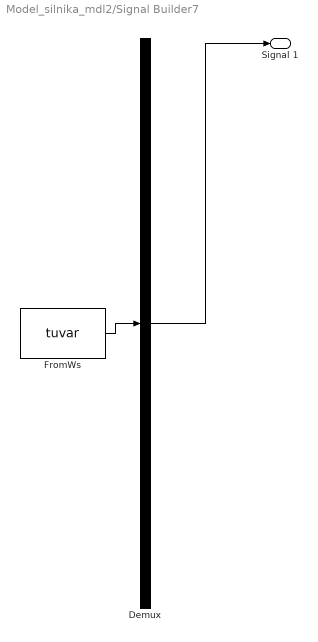
== system Model_silnika_mdl2/Signal Builder7 ==
  Demux : Demux  Tag=STV Demux  Outputs=1
  FromWs : FromWorkspace  Tag=STV FromWs  VariableName=tuvar  SampleTime=0  SigBuilderData=DataTag14  VnvData=DataTag15
      SigBuilderData=|
      | common.afterFinalStr = 'Extrapolate'
      | common.sampleTime = 0
      | dataSet.timeRange = [0 1000]
      | dataSet.name = 'Group 1'
      | sbobj.Groups.Name = 'Group 1'
      | sbobj.Groups.Signals.Name = 'Signal 1'
      | sbobj.Groups.Signals.XData = [0 5 10 40 72 94 1000]
      | sbobj.Groups.Signals.YData = [0 2 2 196 238 246 250]
      | sbobj.Groups.TimeRange = [0 1000]
  Signal 1 : Outport  Tag=STV Outport
  wires:
  Demux/1 -> Signal 1/1
  FromWs/1 -> Demux/1

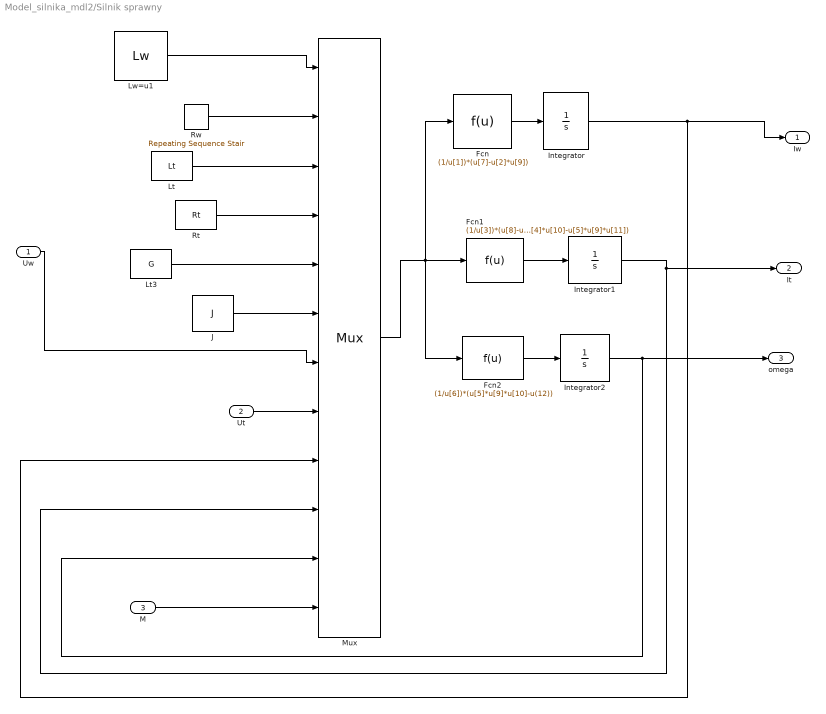
== system Model_silnika_mdl2/Silnik sprawny ==
  Uw : Inport
  Ut : Inport  Port=2
  M : Inport  Port=3
  Fcn : Fcn  Expr=(1/u[1])*(u[7]-u[2]*u[9])  SampleTime=0.25
  Fcn1 : Fcn  Expr=(1/u[3])*(u[8]-u[4]*u[10]-u[5]*u[9]*u[11])
  Fcn2 : Fcn  Expr=(1/u[6])*(u[5]*u[9]*u[10]-u(12))
  Integrator : Integrator
  Integrator1 : Integrator
  Integrator2 : Integrator
  J : Constant  Value=J
  Lt : Constant  Value=Lt
  Lt3 : Constant  Value=G
  Lw=u1 : Constant  Value=Lw
  Mux : Mux  Inputs=12
  Rt : Constant  Value=Rt
  Rw : simulink/Sources/Repeating Sequence Stair  OutValues=Rw  tsamp=0.25  OutMin=[]  OutMax=[]  OutDataTypeStr=double  OutputDataTypeScalingMode=double  OutDataType=fixdt(0,8)  ConRadixGroup=Best Precision: Vector-wise  OutScaling=2^-12
  Iw : Outport
  It : Outport  Port=2
  omega : Outport  Port=3
  wires:
  Lw=u1/1 -> Mux/1
  Lt/1 -> Mux/3
  J/1 -> Mux/6
  Fcn/1 -> Integrator/1
  Fcn1/1 -> Integrator1/1
  Integrator/1 -> Mux/9, Iw/1
  Integrator1/1 -> Mux/10, It/1
  Fcn2/1 -> Integrator2/1
  Integrator2/1 -> Mux/11, omega/1
  Mux/1 -> Fcn2/1, Fcn/1, Fcn1/1
  Uw/1 -> Mux/7
  M/1 -> Mux/12
  Ut/1 -> Mux/8
  Lt3/1 -> Mux/5
  Rw/1 -> Mux/2
  Rt/1 -> Mux/4

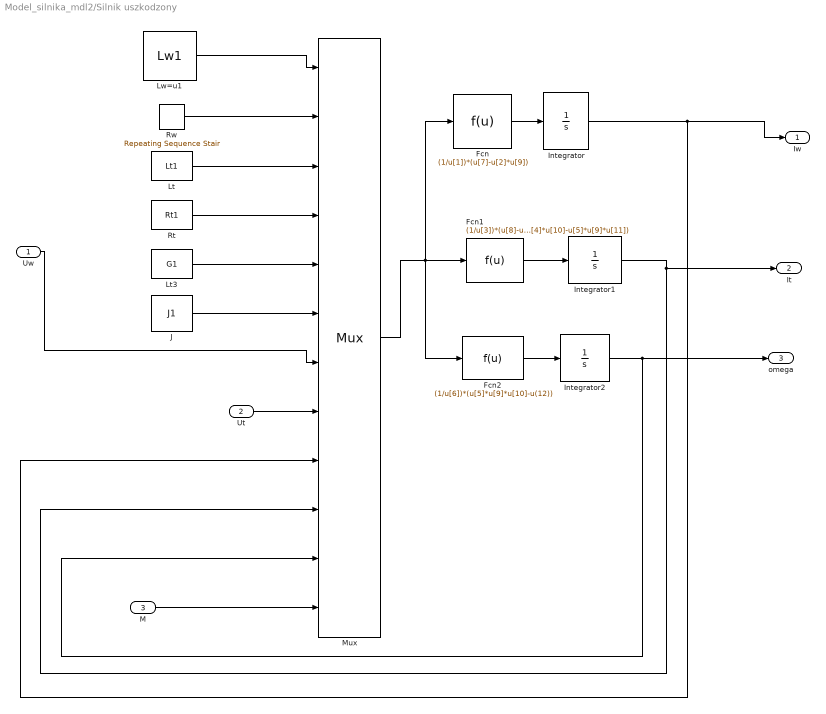
== system Model_silnika_mdl2/Silnik uszkodzony ==
  Uw : Inport
  Ut : Inport  Port=2
  M : Inport  Port=3
  Fcn : Fcn  Expr=(1/u[1])*(u[7]-u[2]*u[9])  SampleTime=0.25
  Fcn1 : Fcn  Expr=(1/u[3])*(u[8]-u[4]*u[10]-u[5]*u[9]*u[11])
  Fcn2 : Fcn  Expr=(1/u[6])*(u[5]*u[9]*u[10]-u(12))
  Integrator : Integrator
  Integrator1 : Integrator
  Integrator2 : Integrator
  J : Constant  Value=J1
  Lt : Constant  Value=Lt1
  Lt3 : Constant  Value=G1
  Lw=u1 : Constant  Value=Lw1
  Mux : Mux  Inputs=12
  Rt : Constant  Value=Rt1
  Rw : simulink/Sources/Repeating Sequence Stair  OutValues=Rw1  tsamp=0.25  OutMin=[]  OutMax=[]  OutDataTypeStr=double  OutputDataTypeScalingMode=double  OutDataType=fixdt(0,8)  ConRadixGroup=Best Precision: Vector-wise  OutScaling=2^-12
  Iw : Outport
  It : Outport  Port=2
  omega : Outport  Port=3
  wires:
  Lw=u1/1 -> Mux/1
  Lt/1 -> Mux/3
  J/1 -> Mux/6
  Fcn/1 -> Integrator/1
  Fcn1/1 -> Integrator1/1
  Integrator/1 -> Mux/9, Iw/1
  Integrator1/1 -> Mux/10, It/1
  Fcn2/1 -> Integrator2/1
  Integrator2/1 -> Mux/11, omega/1
  Mux/1 -> Fcn2/1, Fcn/1, Fcn1/1
  Uw/1 -> Mux/7
  M/1 -> Mux/12
  Ut/1 -> Mux/8
  Lt3/1 -> Mux/5
  Rw/1 -> Mux/2
  Rt/1 -> Mux/4
